simulink model "substation"  (R2018a)
settings: Solver=ode15s  StartTime=0.0  StopTime=0.5  MaxStep=50e-6  RelTol=1e-3  EnableMultiTasking=on
undefined symbols (not defined in the file or in its folder): D1, Delta, Ts
libraries: powerlib x69, powerlib_extras x50
(part 1 of 2)
settings Model: Creator=anton  LastModifiedBy=thain
settings OptimizationCC: LifeSpan=inf
settings DebuggingCC: SFUnexpectedBacktrackingDiag=warning  SFNoUnconditionalDefaultTransitionDiag=warning
settings CodeAppCC: StateflowObjectComments=on
settings GRTTargetCC: TargetLangStandard=C89/C90 (ANSI)
settings ConfigComp: CovMetricSettings=dw  CovSaveCumulativeToWorkspaceVar=on  CovSaveSingleToWorkspaceVar=on  CovExternalEMLEnable=off
settings SimscapeCC: SimscapeNormalizeSystem=off

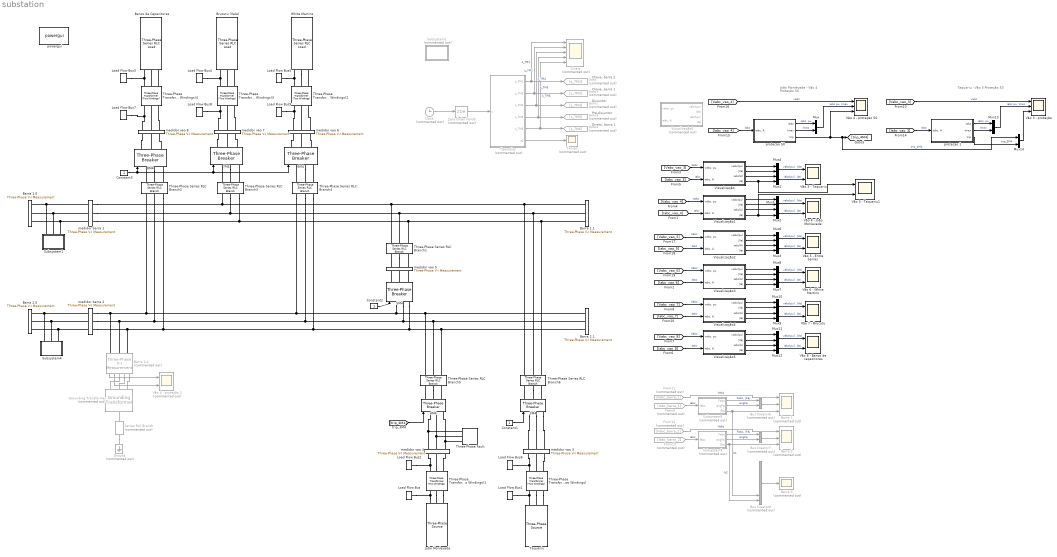
== system substation ==
  note: João Monlevade - Vão 4
      | Proteção 50
  note: Chave, barra 2
  note: Disjuntor
  note: Pré-disjuntor
  note: Chave, barra 1
  note: Direto, barra 1
  note: Taquariu - Vão 3
      | Proteção 50
  3M4 : powerlib/Elements/Three-Phase Breaker  InitialState=closed  SwitchA=on  SwitchB=on  SwitchC=on  SwitchTimes="[1/60  5/60]"  External=on  BreakerResistance=0.01  SnubberResistance=1e6  SnubberCapacitance=inf  Measurements=None
  4M4 : powerlib/Elements/Three-Phase Breaker  InitialState=closed  SwitchA=on  SwitchB=on  SwitchC=on  SwitchTimes="[1/60  5/60]"  External=on  BreakerResistance=0.01  SnubberResistance=1e6  SnubberCapacitance=inf  Measurements=None
  5M4 : powerlib/Elements/Three-Phase Breaker  InitialState=closed  SwitchA=on  SwitchB=on  SwitchC=on  SwitchTimes="[1/60  5/60]"  External=on  BreakerResistance=0.01  SnubberResistance=1e6  SnubberCapacitance=inf  Measurements=None
  6M4 : powerlib/Elements/Three-Phase Breaker  InitialState=closed  SwitchA=on  SwitchB=on  SwitchC=on  SwitchTimes="[1/60  5/60]"  External=on  BreakerResistance=0.01  SnubberResistance=1e6  SnubberCapacitance=inf  Measurements=None
  7M4 : powerlib/Elements/Three-Phase Breaker  InitialState=closed  SwitchA=on  SwitchB=on  SwitchC=on  SwitchTimes="[1/60  5/60]"  External=on  BreakerResistance=0.01  SnubberResistance=1e6  SnubberCapacitance=inf  Measurements=None
  8M4 : powerlib/Elements/Three-Phase Breaker  InitialState=closed  SwitchA=on  SwitchB=on  SwitchC=on  SwitchTimes="[1/60  5/60]"  External=on  BreakerResistance=0.01  SnubberResistance=1e6  SnubberCapacitance=inf  Measurements=None
  Banco de Capacitores : powerlib/Elements/Three-Phase Series RLC Load  LConnTagsString=A|B|C  Configuration=Y (grounded)  NominalVoltage=230e3  Vabc=[1e3 1e3 1e3]  Vabcp=[1e3 1e3 1e3]  NominalFrequency=60  UnbalancedPower=off  ActivePower=capacitor.P  InductivePower=capacitor.QL  CapacitivePower=capacitor.QC  Pabc=[10e3 9e3 11e3]  QLabc=[100 90 110]  QCabc=[100 90 110]  Pabcp=[10e3 9e3 11e3]  QLabcp=[100 90 110]  QCabcp=[100 90 110]  Measurements=None  LoadType=constant Z
  Barra 1 : Scope  Commented=on  NumInputPorts=3
  Barra 1.0 : powerlib/Measurements/Three-Phase V-I Measurement  VoltageMeasurement=no  SetLabelV=off  LabelV=Vabc  Vpu=off  VpuLL=off  CurrentMeasurement=no  SetLabelI=off  LabelI=Iabc  Ipu=off  Pbase=100e6  Vbase=500e3  OutputType=Complex  PhasorSimulation=off  PSBequivalent=0
  Barra 1.1 : powerlib/Measurements/Three-Phase V-I Measurement  VoltageMeasurement=no  SetLabelV=off  LabelV=Vabc  Vpu=off  VpuLL=off  CurrentMeasurement=no  SetLabelI=off  LabelI=Iabc  Ipu=off  Pbase=100e6  Vbase=500e3  OutputType=Complex  PhasorSimulation=off  PSBequivalent=0
  Barra 2 : Scope  Commented=on  NumInputPorts=3
  Barra 2.0 : powerlib/Measurements/Three-Phase V-I Measurement  VoltageMeasurement=no  SetLabelV=off  LabelV=Vabc  Vpu=off  VpuLL=off  CurrentMeasurement=no  SetLabelI=off  LabelI=Iabc  Ipu=off  Pbase=100e6  Vbase=500e3  OutputType=Complex  PhasorSimulation=off  PSBequivalent=0
  Barra 2.1 : powerlib/Measurements/Three-Phase V-I Measurement  VoltageMeasurement=no  SetLabelV=off  LabelV=Vabc  Vpu=off  VpuLL=off  CurrentMeasurement=no  SetLabelI=off  LabelI=Iabc  Ipu=off  Pbase=100e6  Vbase=500e3  OutputType=Complex  PhasorSimulation=off  PSBequivalent=0
  Barra 2.2 : powerlib/Measurements/Three-Phase V-I Measurement  Commented=on  VoltageMeasurement=phase-to-ground  SetLabelV=off  LabelV=Vabc  Vpu=off  VpuLL=off  CurrentMeasurement=yes  SetLabelI=off  LabelI=Iabc  Ipu=off  Pbase=100e6  Vbase=500e3  OutputType=Complex  PhasorSimulation=off  PSBequivalent=0
  Barra 3 : Scope  Commented=on
  Brucutu (Vale) : powerlib/Elements/Three-Phase Series RLC Load  LConnTagsString=A|B|C  Configuration=Y (grounded)  NominalVoltage=230e3  Vabc=[1e3 1e3 1e3]  Vabcp=[1e3 1e3 1e3]  NominalFrequency=60  UnbalancedPower=off  ActivePower=brucutu.P  InductivePower=brucutu.QL  CapacitivePower=brucutu.QC  Pabc=[10e3 9e3 11e3]  QLabc=[100 90 110]  QCabc=[100 90 110]  Pabcp=[10e3 9e3 11e3]  QLabcp=[100 90 110]  QCabcp=[100 90 110]  Measurements=None  LoadType=constant Z
  Bus Creator6 : BusCreator  Commented=on  Inputs=2
  Bus Creator7 : BusCreator  Commented=on  Inputs=2
  Bus Creator8 : BusCreator  Commented=on  Inputs=8
  Clock : Clock  Commented=on
  Constant1 : Constant
  Constant2 : Constant
  Constant3 : Constant
  From11 : From  Commented=on  GotoTag=Vabc_barra_1  TagVisibility=global
  From12 : From  Commented=on  GotoTag=Vabc_barra_2  TagVisibility=global
  From13 : From  Commented=on  GotoTag=Iabc_barra_2  TagVisibility=global
  From9 : From  Commented=on  GotoTag=Iabc_barra_1  TagVisibility=global
  Goto : Goto  Commented=on  GotoTag=s_7M1
  Goto1 : Goto  Commented=on  GotoTag=s_7M2
  Goto2 : Goto  Commented=on  GotoTag=s_7M4
  Goto3 : Goto  Commented=on  GotoTag=s_7M5
  Goto4 : Goto  Commented=on  GotoTag=s_7M6
  Ground : powerlib/Elements/Ground  Commented=on  LConnTagsString=a
  "Grounding Transformer " : powerlib/Elements/Grounding Transformer   Commented=on  UNITS=pu  NominalPower="[1000*100e6   60]"  NominalVoltage=230e3  ZeroSequenceImpedance_pu=[1e-4 1e-4]  MagnetizationBranch_pu=[1e4 1e4]  ZeroSequenceImpedance_SI=[0.052083 589.05]  MagnetizationBranch_SI=[1041.7 3.927e+005]  Measurements=None
      settings: SourceProductName=Simscape Power Systems  SourceProductBaseCode=PS
  João Monlevade : powerlib/Electrical Sources/Three-Phase Source  InternalConnection=Yg  VoltagePhases=off  Voltage=(230000)*1  PhaseAngle=0.0008361  Voltage_phases=[25e3 25e3 25e3]/sqrt(3)  PhaseAngles_phases=[0 -120 +120]  Frequency=60  NonIdealSource=on  SpecifyImpedance=on  Resistance=0  Inductance=0  ShortCircuitLevel=136243*1e6  BaseVoltage=230e3  XRratio=7  BusType=PQ  Pref=monlevade.P  Qref=monlevade.Q  Prefabc=[10e3, 10e3, 10e3]  Qrefabc=[0, 0, 0]  Qmin=-inf  Qmax=inf
  Load Flow Bus : powerlib/Measurements/Load Flow Bus  LConnTagsString=a  Phases=single  Connectors=on one side  ID=BUS_vao4  Vbase=230e3  Vref=1  Vangle=0  VLF=1  VLFb=1  VLFc=1  angleLF=1.025e-06  angleLFb=0  angleLFc=0
      settings: SourceProductName=Simscape Power Systems
  Load Flow Bus1 : powerlib/Measurements/Load Flow Bus  LConnTagsString=a  Phases=single  Connectors=on one side  ID=BUS_vao3  Vbase=230e3  Vref=1  Vangle=0  VLF=1  VLFb=1  VLFc=1  angleLF=0  angleLFb=0  angleLFc=0
      settings: SourceProductName=Simscape Power Systems
  Load Flow Bus2 : powerlib/Measurements/Load Flow Bus  LConnTagsString=a  Phases=single  Connectors=on one side  ID=BUS_vao4_barra  Vbase=230e3  Vref=1  Vangle=0  VLF=1  VLFb=1  VLFc=1  angleLF=-30  angleLFb=0  angleLFc=0
      settings: SourceProductName=Simscape Power Systems
  Load Flow Bus3 : powerlib/Measurements/Load Flow Bus  LConnTagsString=a  Phases=single  Connectors=on one side  ID=BUS_capacitor  Vbase=230e3  Vref=1  Vangle=0  VLF=1  VLFb=1  VLFc=1  angleLF=-7.41e-06  angleLFb=0  angleLFc=0
      settings: SourceProductName=Simscape Power Systems
  Load Flow Bus4 : powerlib/Measurements/Load Flow Bus  LConnTagsString=a  Phases=single  Connectors=on one side  ID=BUS_c2  Vbase=230e3  Vref=1  Vangle=0  VLF=1  VLFb=1  VLFc=1  angleLF=8.861e-06  angleLFb=0  angleLFc=0
      settings: SourceProductName=Simscape Power Systems
  Load Flow Bus5 : powerlib/Measurements/Load Flow Bus  LConnTagsString=a  Phases=single  Connectors=on one side  ID=BUS_c1  Vbase=230e3  Vref=1  Vangle=0  VLF=1  VLFb=1  VLFc=1  angleLF=6.428e-06  angleLFb=0  angleLFc=0
      settings: SourceProductName=Simscape Power Systems
  Load Flow Bus6 : powerlib/Measurements/Load Flow Bus  LConnTagsString=a  Phases=single  Connectors=on one side  ID=BUS_vao3_barra  Vbase=230e3  Vref=1  Vangle=0  VLF=1  VLFb=1  VLFc=1  angleLF=-30  angleLFb=0  angleLFc=0
      settings: SourceProductName=Simscape Power Systems
  Load Flow Bus7 : powerlib/Measurements/Load Flow Bus  LConnTagsString=a  Phases=single  Connectors=on one side  ID=BUS_capacitor_barra  Vbase=230e3  Vref=1  Vangle=0  VLF=1  VLFb=1  VLFc=1  angleLF=-30  angleLFb=0  angleLFc=0
      settings: SourceProductName=Simscape Power Systems
  Load Flow Bus8 : powerlib/Measurements/Load Flow Bus  LConnTagsString=a  Phases=single  Connectors=on one side  ID=BUS_c2_barra  Vbase=230e3  Vref=1  Vangle=0  VLF=1  VLFb=1  VLFc=1  angleLF=-30  angleLFb=0  angleLFc=0
      settings: SourceProductName=Simscape Power Systems
  Load Flow Bus9 : powerlib/Measurements/Load Flow Bus  LConnTagsString=a  Phases=single  Connectors=on one side  ID=BUS_c1_barra  Vbase=230e3  Vref=1  Vangle=0  VLF=1  VLFb=1  VLFc=1  angleLF=-30  angleLFb=0  angleLFc=0
      settings: SourceProductName=Simscape Power Systems
  Mux{,1..14} (15 alike) : Mux  Inputs=2
  Operation : MATLAB Function  Commented=on  TreatAsAtomicUnit=on
  Series RLC Branch : powerlib/Elements/Series RLC Branch  Commented=on  LConnTagsString=__new0  RConnTagsString=__new0  BranchType=R  Resistance=1e12  Inductance=1e-3  SetiL0=off  InitialCurrent=0  Capacitance=1e-6  Setx0=off  InitialVoltage=0  Measurements=None
  Sinais : Scope  Commented=on  NumInputPorts=5
  Subsystem1 : Subsystem
  Subsystem2 : Subsystem  Commented=on
  Subsystem4 : Subsystem
  Subsystem8 : Subsystem  Commented=on
  Subsystem9 : Subsystem  Commented=on
  Taquariu : powerlib/Electrical Sources/Three-Phase Source  InternalConnection=Yg  VoltagePhases=off  Voltage=(230000)*1.00001  PhaseAngle=0.00049007  Voltage_phases=[25e3 25e3 25e3]/sqrt(3)  PhaseAngles_phases=[0 -120 +120]  Frequency=60  NonIdealSource=on  SpecifyImpedance=on  Resistance=0  Inductance=0  ShortCircuitLevel=51788*1e6  BaseVoltage=230e3  XRratio=7  BusType=swing  Pref=11e6  Qref=0  Prefabc=[10e3, 10e3, 10e3]  Qrefabc=[0, 0, 0]  Qmin=-inf  Qmax=inf
  Tempo : Scope  Commented=on
  Three-Phase Series RLC Branch{1..6} (6 alike) : powerlib/Elements/Three-Phase Series RLC Branch  LConnTagsString=A|B|C  RConnTagsString=A|B|C  BranchType=R  Resistance=1e-5  Inductance=1e-3  Capacitance=1e-6  Measurements=None
  Three-Phase Transformer (Two Windings){,1..4} (5 alike) : powerlib/Elements/Three-Phase Transformer (Two Windings)  Winding1Connection=Delta (D1)  Winding2Connection=Yg  CoreType=Three single-phase transformers  SetSaturation=off  Hysteresis=off  DataFile='hysteresis'  SetInitialFlux=off  Measurements=None  UNITS=pu  NominalPower=[ 100e9 , 60 ]  Winding1=[230e3 1e-4 1e-4]  Winding2=[230e3 1e-4 1e-4]  Rm=1e6  Lm=1e6  L0=0.5  Saturation=[0 0;1.8776e-06 3.8348;0.0007823 4.8574]  InitialFluxes=[ 0.8 , -0.8 , 0.7 ]  MoreParameters=off  BreakLoop=off  DataType=off  TransfoNumber=1
  Three-Phase Fault : powerlib/Elements/Three-Phase Fault  InitialStates=0  FaultA=on  FaultB=on  FaultC=on  GroundFault=on  SwitchTimes="[0.1  2+1/60]"  External=off  SwitchStatus=NaN  FaultResistance=0.001  GroundResistance=0.01  SnubberResistance=1e6  SnubberCapacitance=inf  Measurements=None
  Visualização : Subsystem
  Visualização1 : Subsystem
  Visualização2 : Subsystem
  Visualização3 : Subsystem
  Visualização4 : Subsystem
  Visualização5 : Subsystem
  Visualização6 : Subsystem  Commented=on  mask{I_base=2.236}
      mask prompts: I_base "Ibase, A"
  Vão 3 - Taquariu : Scope  NumInputPorts=2
  Vão 3 - Taquariu1 : Scope  NumInputPorts=2
  Vão 3 - proteção : Scope  NumInputPorts=3
  Vão 4 - João Monlevade : Scope  NumInputPorts=2
  Vão 4 - proteção 1 : Scope  Commented=on  NumInputPorts=2
  Vão 4 - proteção 50 : Scope  NumInputPorts=3
  Vão 5 - Entre barras : Scope  NumInputPorts=2
  Vão 6 - White Martins : Scope  NumInputPorts=2
  Vão 7 - Brucutu : Scope  NumInputPorts=2
  Vão 8 - Banco de capacitores : Scope  NumInputPorts=2
  White Martins : powerlib/Elements/Three-Phase Series RLC Load  LConnTagsString=A|B|C  Configuration=Y (grounded)  NominalVoltage=230e3  Vabc=[1e3 1e3 1e3]  Vabcp=[1e3 1e3 1e3]  NominalFrequency=60  UnbalancedPower=off  ActivePower=white.P  InductivePower=white.QL  CapacitivePower=white.QC  Pabc=[10e3 9e3 11e3]  QLabc=[100 90 110]  QCabc=[100 90 110]  Pabcp=[10e3 9e3 11e3]  QLabcp=[100 90 110]  QCabcp=[100 90 110]  Measurements=None  LoadType=constant Z
  Zero-Order Hold3 : ZeroOrderHold  Commented=on  SampleTime=Ts
  medidor barra 1 : powerlib/Measurements/Three-Phase V-I Measurement  VoltageMeasurement=phase-to-ground  SetLabelV=on  LabelV=Vabc_barra_1  Vpu=on  VpuLL=off  CurrentMeasurement=no  SetLabelI=on  LabelI=Iabc_barra_1  Ipu=on  Pbase=16*100e6  Vbase=230e3  OutputType=Complex  PhasorSimulation=off  PSBequivalent=0
  medidor barra 2 : powerlib/Measurements/Three-Phase V-I Measurement  VoltageMeasurement=phase-to-ground  SetLabelV=on  LabelV=Vabc_barra_2  Vpu=on  VpuLL=off  CurrentMeasurement=no  SetLabelI=on  LabelI=Iabc_barra_2  Ipu=off  Pbase=100e6  Vbase=230e3  OutputType=Complex  PhasorSimulation=off  PSBequivalent=0
  medidor vao 3 : powerlib/Measurements/Three-Phase V-I Measurement  VoltageMeasurement=phase-to-ground  SetLabelV=on  LabelV=Vabc_vao_3  Vpu=on  VpuLL=off  CurrentMeasurement=yes  SetLabelI=on  LabelI=Iabc_vao_3  Ipu=off  Pbase=16*100e6  Vbase=230e3  OutputType=Complex  PhasorSimulation=off  PSBequivalent=0
  medidor vao 4 : powerlib/Measurements/Three-Phase V-I Measurement  VoltageMeasurement=phase-to-ground  SetLabelV=on  LabelV=Vabc_vao_4  Vpu=on  VpuLL=off  CurrentMeasurement=yes  SetLabelI=on  LabelI=Iabc_vao_4  Ipu=off  Pbase=16*100e6  Vbase=230e3  OutputType=Complex  PhasorSimulation=off  PSBequivalent=0
  medidor vao 5 : powerlib/Measurements/Three-Phase V-I Measurement  VoltageMeasurement=phase-to-ground  SetLabelV=on  LabelV=Vabc_vao_5  Vpu=on  VpuLL=off  CurrentMeasurement=yes  SetLabelI=on  LabelI=Iabc_vao_5  Ipu=off  Pbase=16*100e6  Vbase=230e3  OutputType=Complex  PhasorSimulation=off  PSBequivalent=0
  medidor vao 6 : powerlib/Measurements/Three-Phase V-I Measurement  VoltageMeasurement=phase-to-ground  SetLabelV=on  LabelV=Vabc_vao_6  Vpu=on  VpuLL=off  CurrentMeasurement=yes  SetLabelI=on  LabelI=Iabc_vao_6  Ipu=off  Pbase=16*100e6  Vbase=230e3  OutputType=Complex  PhasorSimulation=off  PSBequivalent=0
  medidor vao 7 : powerlib/Measurements/Three-Phase V-I Measurement  VoltageMeasurement=phase-to-ground  SetLabelV=on  LabelV=Vabc_vao_7  Vpu=on  VpuLL=off  CurrentMeasurement=yes  SetLabelI=on  LabelI=Iabc_vao_7  Ipu=off  Pbase=16*100e6  Vbase=230e3  OutputType=Complex  PhasorSimulation=off  PSBequivalent=0
  medidor vao 8 : powerlib/Measurements/Three-Phase V-I Measurement  VoltageMeasurement=phase-to-ground  SetLabelV=on  LabelV=Vabc_vao_8  Vpu=on  VpuLL=off  CurrentMeasurement=yes  SetLabelI=on  LabelI=Iabc_vao_8  Ipu=off  Pbase=16*100e6  Vbase=230e3  OutputType=Complex  PhasorSimulation=off  PSBequivalent=0
  powergui : powerlib/powergui  Priority=1  SimulationMode=Discrete  SampleTime=25e-6  frequency=60  Iterations=50  frequencyindice=60  Pbase=100e6  ErrMax=0.0001  UnitsV=kV  UnitsW=MW  buscounter=4  FunctionMessages=off  echomessages=off  EnableUseOfTLC=off  CurrentSourceSwitches=off  DisableSnubberDevices=off  DisableRonSwitches=off  DisableVfSwitches=off  DisplayEquations=off  SolverType=Tustin/Backward Euler (TBE)  Interpol=off  ExternalGateDelay=off  methode=off  Ts=100  x0status=blocks  SPID=off  SwTol=0  HookPort=off  RestoreLinks=warning  ResistiveCurrentMeasurement=off  Frange=[0:2:500]  Ylog=off  Xlog=on  ShowGrid=off  save=off  variable=ZData  structure=0  ZoomFFT=off  StartTime=0.0  cycles=1  DisplayStyle=1  fundamental=60  FreqAxis=off  MaxFrequency=1000  frequencyindicesteady=1  RmsSteady=1  display=off
  protecao 1 : Subsystem  mask{Ipick_up=0*6.8 + 4.8e5/2, td_op=1.0*(1/60)}
      mask prompts: Ipick_up "Ipick-up, A"; td_op "delay de operação, s"
  protecao 50 : Subsystem  mask{Ipick_up=0*6.8 + 4.8e5/2, td_op=1.0*(1/60)}
      mask prompts: Ipick_up "Ipick-up, A"; td_op "delay de operação, s"
  wires:
  Operation/5(s_7M6) -> Sinais/5, Goto4/1  "s_7M6"
  Operation/6(t0) -> Tempo/1
  Operation/4(s_7M5) -> Sinais/4, Goto3/1  "s_7M5"
  Operation/2(s_7M2) -> Sinais/2, Goto1/1  "s_7M2"
  Zero-Order Hold3/1 -> Operation/1(t)
  Operation/3(s_7M4) -> Sinais/3, Goto2/1  "s_7M4"
  Clock/1 -> Zero-Order Hold3/1
  Operation/1(s_7M1) -> Sinais/1, Goto/1  "s_7M1"
  Constant2/1 -> 5M4/1
  Constant3/1 -> 6M4/1, 7M4/1, 8M4/1
  Bus Creator6/1 -> Barra 1/2
  Subsystem8/3(|Fa|) -> Bus Creator8/7, Barra 1/3  "b1"
  Subsystem8/2(angFa) -> Bus Creator6/2  "angFa"
  Subsystem8/1(Fabc) -> Bus Creator6/1  "Fabc, |Fa|"
  From9/1 -> Subsystem8/1(fabc)  "Iabc"
  From11/1 -> Barra 1/1  "Vabc"
  From12/1 -> Barra 2/1  "Vabc"
  From13/1 -> Subsystem9/1(fabc)  "Iabc"
  Subsystem9/1(Fabc) -> Bus Creator7/1  "Fabc, |Fa|"
  Subsystem9/2(angFa) -> Bus Creator7/2  "angFa"
  Subsystem9/3(|Fa|) -> Bus Creator8/8, Barra 2/3  "b2"
  Bus Creator7/1 -> Barra 2/2
  Bus Creator8/1 -> Barra 3/1
  protecao 50/3(trip) -> Mux14/1, [trip_4M4], Vão 4 - proteção 50/3  "trip_4M4"
  protecao 50/1(iabc) -> Mux/1  "iabc, pu"
  Mux/1 -> Vão 4 - proteção 50/2  "iabc pu, Imax"
  [Iabc_vao_4] -> protecao 50/1("iabc, A")  "Iabc"
  protecao 50/2(Imax) -> Mux/2  "Imax"
  [Vabc_vao_4] -> Vão 4 - proteção 50/1  "vabc"
  [Vabc_vao_3] -> Visualização/1("vabc, pu")  "Vabc"
  [Iabc_vao_3] -> Visualização/2("iabc, A")  "Iabc"
  Mux4/1 -> Vão 3 - Taquariu/1  "vabc(pu), |Va|"
  Mux1/1 -> Vão 3 - Taquariu/2  "iabc(pu), |Ia|"
  Visualização/4(|Ia|) -> Vão 3 - Taquariu1/1, Mux1/2
  Visualização/3(iabc(A)) -> Mux1/1
  [Iabc_vao_4] -> Visualização1/2("iabc, A")  "Iabc"
  [Vabc_vao_4] -> Visualização1/1("vabc, pu")  "Vabc"
  [Vabc_vao_5] -> Visualização2/1("vabc, pu")  "Vabc"
  [Iabc_vao_5] -> Visualização2/2("iabc, A")  "Iabc"
  Visualização/1(vabc(pu)) -> Mux4/1
  Visualização/2(|Va|) -> Mux4/2
  Visualização1/2(|Va|) -> Mux5/2
  Visualização1/1(vabc(pu)) -> Mux5/1
  Visualização1/3(iabc(A)) -> Mux2/1
  Visualização1/4(|Ia|) -> Vão 3 - Taquariu1/2, Mux2/2
  Mux2/1 -> Vão 4 - João Monlevade/2  "iabc(pu), |Ia|"
  Mux5/1 -> Vão 4 - João Monlevade/1  "vabc(pu), |Va|"
  Mux6/1 -> Vão 5 - Entre barras/1  "vabc(pu), |Va|"
  Mux3/1 -> Vão 5 - Entre barras/2  "iabc(pu), |Ia|"
  Visualização2/4(|Ia|) -> Mux3/2
  Visualização2/3(iabc(A)) -> Mux3/1
  Visualização2/1(vabc(pu)) -> Mux6/1
  Visualização2/2(|Va|) -> Mux6/2
  Visualização3/2(|Va|) -> Mux8/2
  Visualização3/1(vabc(pu)) -> Mux8/1
  Visualização3/3(iabc(A)) -> Mux7/1
  Visualização3/4(|Ia|) -> Mux7/2
  Mux7/1 -> Vão 6 - White Martins/2  "iabc(pu), |Ia|"
  Mux8/1 -> Vão 6 - White Martins/1  "vabc(pu), |Va|"
  [Iabc_vao_6] -> Visualização3/2("iabc, A")  "Iabc"
  [Vabc_vao_6] -> Visualização3/1("vabc, pu")  "Vabc"
  [Vabc_vao_7] -> Visualização4/1("vabc, pu")  "Vabc"
  [Iabc_vao_7] -> Visualização4/2("iabc, A")  "Iabc"
  Mux10/1 -> Vão 7 - Brucutu/1  "vabc(pu), |Va|"
  Mux9/1 -> Vão 7 - Brucutu/2  "iabc(pu), |Ia|"
  Visualização4/4(|Ia|) -> Mux9/2
  Visualização4/3(iabc(A)) -> Mux9/1
  Visualização4/1(vabc(pu)) -> Mux10/1
  Visualização4/2(|Va|) -> Mux10/2
  Visualização5/2(|Va|) -> Mux11/2
  Visualização5/1(vabc(pu)) -> Mux11/1
  Visualização5/3(iabc(A)) -> Mux12/1
  Visualização5/4(|Ia|) -> Mux12/2
  Mux12/1 -> Vão 8 - Banco de capacitores/2  "iabc(pu), |Ia|"
  Mux11/1 -> Vão 8 - Banco de capacitores/1  "vabc(pu), |Va|"
  [Iabc_vao_8] -> Visualização5/2("iabc, A")  "Iabc"
  [Vabc_vao_8] -> Visualização5/1("vabc, pu")  "Vabc"
  Barra 2.2/1 -> Vão 4 - proteção 1/1
  Barra 2.2/2 -> Vão 4 - proteção 1/2
  Constant1/1 -> 3M4/1
  [trip_4M4] -> 4M4/1
  [Vabc_vao_3] -> Vão 3 - proteção/1  "vabc"
  protecao 1/2(Imax) -> Mux13/2  "Imax"
  [Iabc_vao_3] -> protecao 1/1("iabc, A")  "Iabc"
  Mux13/1 -> Vão 3 - proteção/2  "iabc pu, Imax"
  protecao 1/1(iabc) -> Mux13/1  "iabc, pu"
  protecao 1/3(trip) -> Mux14/2  "trip_3M4"
  Mux14/1 -> Vão 3 - proteção/3
  connections:
  medidor barra 2/RConn3 -- Barra 2.2/LConn3 -- Three-Phase Series RLC Branch2/LConn3 -- Three-Phase Series RLC Branch4/LConn3 -- 5M4/LConn3 -- Barra 2.1/LConn3 -- Three-Phase Series RLC Branch5/RConn3
  5M4/RConn1 -- medidor vao 5/RConn1
  5M4/RConn2 -- medidor vao 5/RConn2
  5M4/RConn3 -- medidor vao 5/RConn3
  medidor barra 1/LConn3 -- Subsystem1/LConn3 -- Barra 1.0/RConn3
  medidor barra 1/LConn2 -- Subsystem1/LConn2 -- Barra 1.0/RConn2
  medidor barra 1/LConn1 -- Subsystem1/LConn1 -- Barra 1.0/RConn1
  medidor barra 2/LConn3 -- Subsystem4/LConn3 -- Barra 2.0/RConn3
  medidor barra 2/LConn2 -- Subsystem4/LConn2 -- Barra 2.0/RConn2
  Load Flow Bus2/LConn1 -- medidor vao 4/RConn1 -- Three-Phase Transformer (Two Windings)1/LConn1
  Load Flow Bus6/LConn1 -- medidor vao 3/RConn1 -- Three-Phase Transformer (Two Windings)/LConn1
  Three-Phase Transformer (Two Windings)/RConn2 -- Taquariu/RConn2
  Taquariu/RConn1 -- Three-Phase Transformer (Two Windings)/RConn1 -- Load Flow Bus1/LConn1
  Three-Phase Transformer (Two Windings)/RConn3 -- Taquariu/RConn3
  João Monlevade/RConn1 -- Three-Phase Transformer (Two Windings)1/RConn1 -- Load Flow Bus/LConn1
  Three-Phase Transformer (Two Windings)1/RConn2 -- João Monlevade/RConn2
  Three-Phase Transformer (Two Windings)1/RConn3 -- João Monlevade/RConn3
  Three-Phase Transformer (Two Windings)2/RConn1 -- Load Flow Bus5/LConn1 -- White Martins/LConn1
  White Martins/LConn2 -- Three-Phase Transformer (Two Windings)2/RConn2
  Three-Phase Transformer (Two Windings)2/RConn3 -- White Martins/LConn3
  Load Flow Bus9/LConn1 -- medidor vao 6/LConn1 -- Three-Phase Transformer (Two Windings)2/LConn1
  Three-Phase Transformer (Two Windings)3/RConn2 -- Brucutu (Vale)/LConn2
  Three-Phase Transformer (Two Windings)3/RConn1 -- Load Flow Bus4/LConn1 -- Brucutu (Vale)/LConn1
  Three-Phase Transformer (Two Windings)3/RConn3 -- Brucutu (Vale)/LConn3
  Load Flow Bus8/LConn1 -- medidor vao 7/LConn1 -- Three-Phase Transformer (Two Windings)3/LConn1
  Three-Phase Transformer (Two Windings)4/RConn2 -- Banco de Capacitores/LConn2
  Three-Phase Transformer (Two Windings)4/RConn1 -- Load Flow Bus3/LConn1 -- Banco de Capacitores/LConn1
  Three-Phase Transformer (Two Windings)4/RConn3 -- Banco de Capacitores/LConn3
  Load Flow Bus7/LConn1 -- medidor vao 8/LConn1 -- Three-Phase Transformer (Two Windings)4/LConn1
  medidor barra 2/RConn1 -- Barra 2.2/LConn1 -- Three-Phase Series RLC Branch2/LConn1 -- Three-Phase Series RLC Branch4/LConn1 -- 5M4/LConn1 -- Barra 2.1/LConn1 -- Three-Phase Series RLC Branch5/RConn1
  medidor barra 2/RConn2 -- Barra 2.2/LConn2 -- Three-Phase Series RLC Branch2/LConn2 -- Three-Phase Series RLC Branch4/LConn2 -- 5M4/LConn2 -- Barra 2.1/LConn2 -- Three-Phase Series RLC Branch5/RConn2
  medidor barra 1/RConn1 -- Three-Phase Series RLC Branch3/LConn1 -- Three-Phase Series RLC Branch1/RConn1 -- Three-Phase Series RLC Branch6/RConn1 -- Barra 1.1/LConn1
  medidor barra 1/RConn2 -- Three-Phase Series RLC Branch3/LConn2 -- Three-Phase Series RLC Branch1/RConn2 -- Three-Phase Series RLC Branch6/RConn2 -- Barra 1.1/LConn2
  medidor barra 1/RConn3 -- Three-Phase Series RLC Branch1/RConn3 -- Three-Phase Series RLC Branch6/RConn3 -- Barra 1.1/LConn3 -- Three-Phase Series RLC Branch3/LConn3
  medidor vao 5/LConn1 -- Three-Phase Series RLC Branch1/LConn1
  Three-Phase Series RLC Branch1/LConn2 -- medidor vao 5/LConn2
  medidor vao 5/LConn3 -- Three-Phase Series RLC Branch1/LConn3
  3M4/RConn1 -- Three-Phase Series RLC Branch6/LConn1
  Three-Phase Series RLC Branch6/LConn2 -- 3M4/RConn2
  3M4/RConn3 -- Three-Phase Series RLC Branch6/LConn3
  3M4/LConn2 -- medidor vao 3/LConn2
  3M4/LConn1 -- medidor vao 3/LConn1
  3M4/LConn3 -- medidor vao 3/LConn3
  medidor vao 3/RConn3 -- Three-Phase Transformer (Two Windings)/LConn3
  Three-Phase Transformer (Two Windings)/LConn2 -- medidor vao 3/RConn2
  4M4/RConn1 -- Three-Phase Series RLC Branch5/LConn1
  Three-Phase Series RLC Branch5/LConn2 -- 4M4/RConn2
  4M4/RConn3 -- Three-Phase Series RLC Branch5/LConn3
  medidor vao 4/RConn3 -- Three-Phase Transformer (Two Windings)1/LConn3
  Three-Phase Transformer (Two Windings)1/LConn2 -- medidor vao 4/RConn2
  medidor vao 4/LConn2 -- Three-Phase Fault/LConn2 -- 4M4/LConn2
  medidor vao 4/LConn3 -- Three-Phase Fault/LConn3 -- 4M4/LConn3
  medidor vao 4/LConn1 -- Three-Phase Fault/LConn1 -- 4M4/LConn1
  Three-Phase Series RLC Branch4/RConn1 -- 6M4/LConn1
  6M4/LConn2 -- Three-Phase Series RLC Branch4/RConn2
  Three-Phase Series RLC Branch4/RConn3 -- 6M4/LConn3
  Three-Phase Series RLC Branch3/RConn1 -- 7M4/LConn1
  7M4/LConn2 -- Three-Phase Series RLC Branch3/RConn2
  Three-Phase Series RLC Branch3/RConn3 -- 7M4/LConn3
  Three-Phase Series RLC Branch2/RConn1 -- 8M4/LConn1
  8M4/LConn2 -- Three-Phase Series RLC Branch2/RConn2
  Three-Phase Series RLC Branch2/RConn3 -- 8M4/LConn3
  8M4/RConn2 -- medidor vao 8/RConn2
  8M4/RConn1 -- medidor vao 8/RConn1
  8M4/RConn3 -- medidor vao 8/RConn3
  7M4/RConn2 -- medidor vao 7/RConn2
  7M4/RConn1 -- medidor vao 7/RConn1
  7M4/RConn3 -- medidor vao 7/RConn3
  6M4/RConn2 -- medidor vao 6/RConn2
  6M4/RConn1 -- medidor vao 6/RConn1
  6M4/RConn3 -- medidor vao 6/RConn3
  medidor vao 8/LConn3 -- Three-Phase Transformer (Two Windings)4/LConn3
  medidor vao 8/LConn2 -- Three-Phase Transformer (Two Windings)4/LConn2
  medidor vao 7/LConn3 -- Three-Phase Transformer (Two Windings)3/LConn3
  medidor vao 7/LConn2 -- Three-Phase Transformer (Two Windings)3/LConn2
  medidor vao 6/LConn3 -- Three-Phase Transformer (Two Windings)2/LConn3
  medidor vao 6/LConn2 -- Three-Phase Transformer (Two Windings)2/LConn2
  Barra 2.2/RConn1 -- "Grounding Transformer "/LConn1
  Barra 2.2/RConn2 -- "Grounding Transformer "/LConn2
  Barra 2.2/RConn3 -- "Grounding Transformer "/LConn3
  Series RLC Branch/RConn1 -- Ground/LConn1
  Series RLC Branch/LConn1 -- "Grounding Transformer "/RConn1
  medidor barra 2/LConn1 -- Subsystem4/LConn1 -- Barra 2.0/RConn1

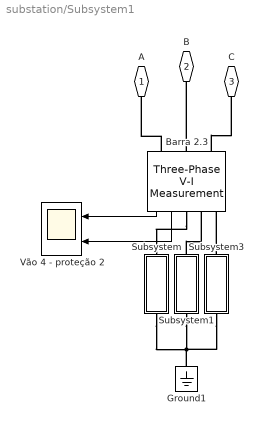
== system substation/Subsystem1 ==
  Barra 2.3 : powerlib/Measurements/Three-Phase V-I Measurement  VoltageMeasurement=phase-to-ground  SetLabelV=off  LabelV=Vabc  Vpu=off  VpuLL=off  CurrentMeasurement=yes  SetLabelI=off  LabelI=Iabc  Ipu=off  Pbase=100e6  Vbase=500e3  OutputType=Complex  PhasorSimulation=off  PSBequivalent=0
  Ground1 : powerlib/Elements/Ground  LConnTagsString=a
  Subsystem : Subsystem
  Subsystem1 : Subsystem
  Subsystem3 : Subsystem
  Vão 4 - proteção 2 : Scope  NumInputPorts=2
  A : PMIOPort  Side=Left
  B : PMIOPort  Port=2  Side=Left
  C : PMIOPort  Port=3  Side=Left
  wires:
  Barra 2.3/1 -> Vão 4 - proteção 2/1
  Barra 2.3/2 -> Vão 4 - proteção 2/2
  connections:
  Barra 2.3/LConn2 -- B/RConn1
  Barra 2.3/LConn3 -- C/RConn1
  Barra 2.3/RConn1 -- Subsystem/LConn1
  Subsystem3/RConn1 -- Ground1/LConn1 -- Subsystem/RConn1 -- Subsystem1/RConn1
  Subsystem1/LConn1 -- Barra 2.3/RConn2
  Subsystem3/LConn1 -- Barra 2.3/RConn3
  Barra 2.3/LConn1 -- A/RConn1

== system substation/Subsystem2 ==
  AC Voltage Source : powerlib/Electrical Sources/AC Voltage Source  Amplitude=sqrt(2)*230e3  Phase=-120  Frequency=60  SampleTime=0  Measurements=None  BusType=swing  Pref=10e3  Qref=0  Qmin=-inf  Qmax=+inf
  AC Voltage Source1 : powerlib/Electrical Sources/AC Voltage Source  Amplitude=sqrt(2)*230e3  Phase=0  Frequency=60  SampleTime=0  Measurements=None  BusType=swing  Pref=10e3  Qref=0  Qmin=-inf  Qmax=+inf
  AC Voltage Source2 : powerlib/Electrical Sources/AC Voltage Source  Amplitude=sqrt(2)*230e3  Phase=120  Frequency=60  SampleTime=0  Measurements=None  BusType=swing  Pref=10e3  Qref=0  Qmin=-inf  Qmax=+inf
  A : PMIOPort  Side=Left
  B : PMIOPort  Port=2  Side=Left
  C : PMIOPort  Port=3  Side=Left
  connections:
  AC Voltage Source1/RConn1 -- A/RConn1 -- AC Voltage Source2/LConn1
  AC Voltage Source/LConn1 -- C/RConn1 -- AC Voltage Source2/RConn1
  AC Voltage Source1/LConn1 -- B/RConn1 -- AC Voltage Source/RConn1

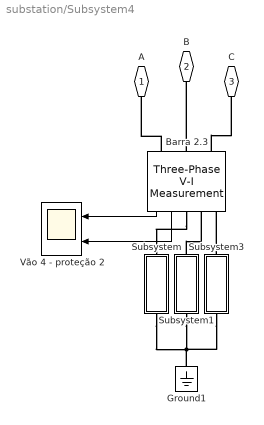
== system substation/Subsystem4 ==
  Barra 2.3 : powerlib/Measurements/Three-Phase V-I Measurement  VoltageMeasurement=phase-to-ground  SetLabelV=off  LabelV=Vabc  Vpu=off  VpuLL=off  CurrentMeasurement=yes  SetLabelI=off  LabelI=Iabc  Ipu=off  Pbase=100e6  Vbase=500e3  OutputType=Complex  PhasorSimulation=off  PSBequivalent=0
  Ground1 : powerlib/Elements/Ground  LConnTagsString=a
  Subsystem : Subsystem
  Subsystem1 : Subsystem
  Subsystem3 : Subsystem
  Vão 4 - proteção 2 : Scope  NumInputPorts=2
  A : PMIOPort  Side=Left
  B : PMIOPort  Port=2  Side=Left
  C : PMIOPort  Port=3  Side=Left
  wires:
  Barra 2.3/2 -> Vão 4 - proteção 2/2
  Barra 2.3/1 -> Vão 4 - proteção 2/1
  connections:
  Barra 2.3/LConn1 -- A/RConn1
  Subsystem3/LConn1 -- Barra 2.3/RConn3
  Subsystem1/LConn1 -- Barra 2.3/RConn2
  Ground1/LConn1 -- Subsystem3/RConn1 -- Subsystem1/RConn1 -- Subsystem/RConn1
  Barra 2.3/RConn1 -- Subsystem/LConn1
  Barra 2.3/LConn3 -- C/RConn1
  Barra 2.3/LConn2 -- B/RConn1

== system substation/Subsystem8 ==
  fabc : Inport
  Demux1 : Demux  Outputs=3
  RMS : powerlib_extras/Measurements/Fourier  f1=60  n=1
  Terminator : Terminator
  Terminator1 : Terminator
  Fabc : Outport
  angFa : Outport  Port=2
  |Fa| : Outport  Port=3
  wires:
  Demux1/2 -> Terminator/1
  Demux1/1 -> RMS/1
  fabc/1 -> Demux1/1, Fabc/1
  RMS/1 -> |Fa|/1  "|fa|"
  RMS/2 -> angFa/1  "angIa"
  Demux1/3 -> Terminator1/1

== system substation/Subsystem9 ==
  fabc : Inport
  Demux1 : Demux  Outputs=3
  RMS : powerlib_extras/Measurements/Fourier  f1=60  n=1
  Terminator : Terminator
  Terminator1 : Terminator
  Fabc : Outport
  angFa : Outport  Port=2
  |Fa| : Outport  Port=3
  wires:
  Demux1/3 -> Terminator1/1
  RMS/2 -> angFa/1  "angIa"
  RMS/1 -> |Fa|/1  "|fa|"
  fabc/1 -> Fabc/1, Demux1/1
  Demux1/1 -> RMS/1
  Demux1/2 -> Terminator/1

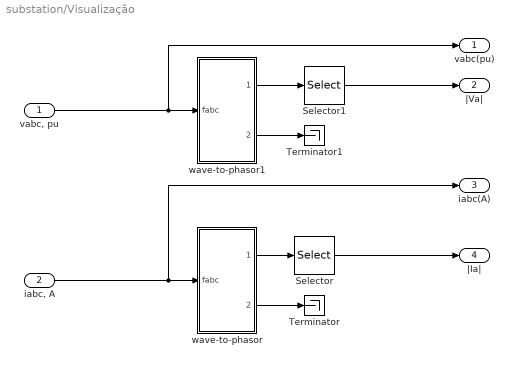
== system substation/Visualização ==
  "vabc, pu" : Inport
  "iabc, A" : Inport  Port=2
  Selector : Selector  InputPortWidth=3  IndexOptions=Index vector (dialog)  Indices=[1]  OutputSizes=1
  Selector1 : Selector  InputPortWidth=3  IndexOptions=Index vector (dialog)  Indices=[1]  OutputSizes=1
  Terminator : Terminator
  Terminator1 : Terminator
  wave-to-phasor : Subsystem
  wave-to-phasor1 : Subsystem
  vabc(pu) : Outport
  |Va| : Outport  Port=2
  iabc(A) : Outport  Port=3
  |Ia| : Outport  Port=4
  wires:
  wave-to-phasor/2(ang(Fabc)) -> Terminator/1
  wave-to-phasor/1(|Fabc|) -> Selector/1
  Selector/1 -> |Ia|/1
  "iabc, A"/1 -> iabc(A)/1, wave-to-phasor/1(fabc)
  "vabc, pu"/1 -> vabc(pu)/1, wave-to-phasor1/1(fabc)
  Selector1/1 -> |Va|/1
  wave-to-phasor1/1(|Fabc|) -> Selector1/1
  wave-to-phasor1/2(ang(Fabc)) -> Terminator1/1

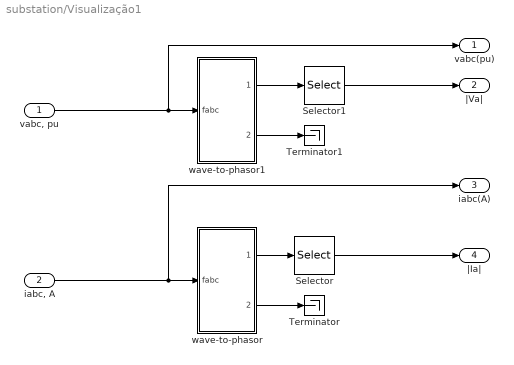
== system substation/Visualização1 ==
  "vabc, pu" : Inport
  "iabc, A" : Inport  Port=2
  Selector : Selector  InputPortWidth=3  IndexOptions=Index vector (dialog)  Indices=[1]  OutputSizes=1
  Selector1 : Selector  InputPortWidth=3  IndexOptions=Index vector (dialog)  Indices=[1]  OutputSizes=1
  Terminator : Terminator
  Terminator1 : Terminator
  wave-to-phasor : Subsystem
  wave-to-phasor1 : Subsystem
  vabc(pu) : Outport
  |Va| : Outport  Port=2
  iabc(A) : Outport  Port=3
  |Ia| : Outport  Port=4
  wires:
  wave-to-phasor1/2(ang(Fabc)) -> Terminator1/1
  wave-to-phasor1/1(|Fabc|) -> Selector1/1
  Selector1/1 -> |Va|/1
  "vabc, pu"/1 -> wave-to-phasor1/1(fabc), vabc(pu)/1
  "iabc, A"/1 -> wave-to-phasor/1(fabc), iabc(A)/1
  Selector/1 -> |Ia|/1
  wave-to-phasor/1(|Fabc|) -> Selector/1
  wave-to-phasor/2(ang(Fabc)) -> Terminator/1

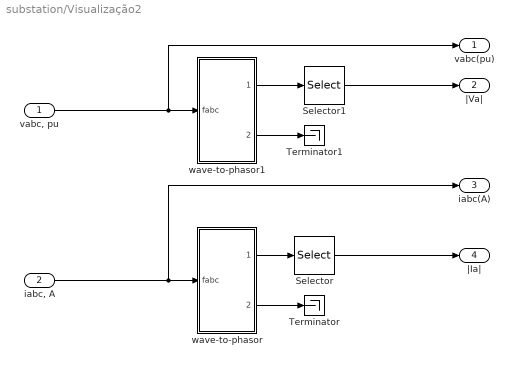
== system substation/Visualização2 ==
  "vabc, pu" : Inport
  "iabc, A" : Inport  Port=2
  Selector : Selector  InputPortWidth=3  IndexOptions=Index vector (dialog)  Indices=[1]  OutputSizes=1
  Selector1 : Selector  InputPortWidth=3  IndexOptions=Index vector (dialog)  Indices=[1]  OutputSizes=1
  Terminator : Terminator
  Terminator1 : Terminator
  wave-to-phasor : Subsystem
  wave-to-phasor1 : Subsystem
  vabc(pu) : Outport
  |Va| : Outport  Port=2
  iabc(A) : Outport  Port=3
  |Ia| : Outport  Port=4
  wires:
  wave-to-phasor/2(ang(Fabc)) -> Terminator/1
  wave-to-phasor/1(|Fabc|) -> Selector/1
  Selector/1 -> |Ia|/1
  "iabc, A"/1 -> iabc(A)/1, wave-to-phasor/1(fabc)
  "vabc, pu"/1 -> vabc(pu)/1, wave-to-phasor1/1(fabc)
  Selector1/1 -> |Va|/1
  wave-to-phasor1/1(|Fabc|) -> Selector1/1
  wave-to-phasor1/2(ang(Fabc)) -> Terminator1/1

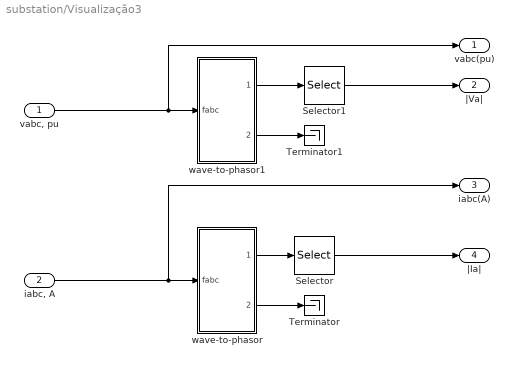
== system substation/Visualização3 ==
  "vabc, pu" : Inport
  "iabc, A" : Inport  Port=2
  Selector : Selector  InputPortWidth=3  IndexOptions=Index vector (dialog)  Indices=[1]  OutputSizes=1
  Selector1 : Selector  InputPortWidth=3  IndexOptions=Index vector (dialog)  Indices=[1]  OutputSizes=1
  Terminator : Terminator
  Terminator1 : Terminator
  wave-to-phasor : Subsystem
  wave-to-phasor1 : Subsystem
  vabc(pu) : Outport
  |Va| : Outport  Port=2
  iabc(A) : Outport  Port=3
  |Ia| : Outport  Port=4
  wires:
  wave-to-phasor1/2(ang(Fabc)) -> Terminator1/1
  wave-to-phasor1/1(|Fabc|) -> Selector1/1
  Selector1/1 -> |Va|/1
  "vabc, pu"/1 -> wave-to-phasor1/1(fabc), vabc(pu)/1
  "iabc, A"/1 -> wave-to-phasor/1(fabc), iabc(A)/1
  Selector/1 -> |Ia|/1
  wave-to-phasor/1(|Fabc|) -> Selector/1
  wave-to-phasor/2(ang(Fabc)) -> Terminator/1

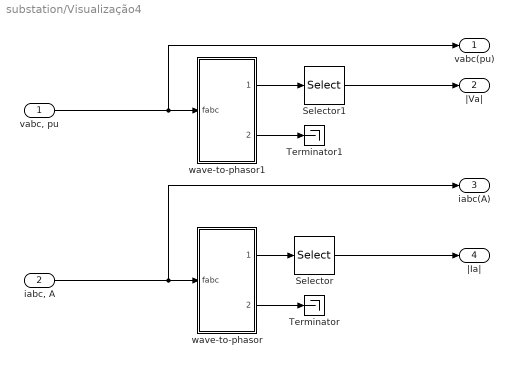
== system substation/Visualização4 ==
  "vabc, pu" : Inport
  "iabc, A" : Inport  Port=2
  Selector : Selector  InputPortWidth=3  IndexOptions=Index vector (dialog)  Indices=[1]  OutputSizes=1
  Selector1 : Selector  InputPortWidth=3  IndexOptions=Index vector (dialog)  Indices=[1]  OutputSizes=1
  Terminator : Terminator
  Terminator1 : Terminator
  wave-to-phasor : Subsystem
  wave-to-phasor1 : Subsystem
  vabc(pu) : Outport
  |Va| : Outport  Port=2
  iabc(A) : Outport  Port=3
  |Ia| : Outport  Port=4
  wires:
  wave-to-phasor/2(ang(Fabc)) -> Terminator/1
  wave-to-phasor/1(|Fabc|) -> Selector/1
  Selector/1 -> |Ia|/1
  "iabc, A"/1 -> iabc(A)/1, wave-to-phasor/1(fabc)
  "vabc, pu"/1 -> vabc(pu)/1, wave-to-phasor1/1(fabc)
  Selector1/1 -> |Va|/1
  wave-to-phasor1/1(|Fabc|) -> Selector1/1
  wave-to-phasor1/2(ang(Fabc)) -> Terminator1/1

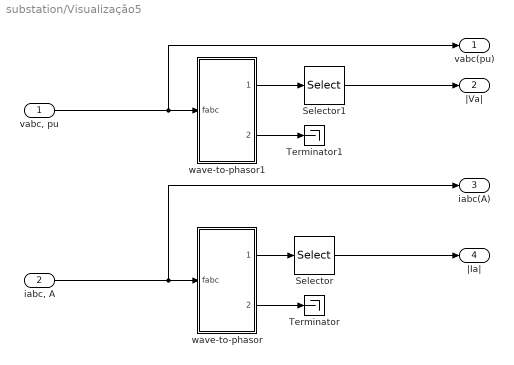
== system substation/Visualização5 ==
  "vabc, pu" : Inport
  "iabc, A" : Inport  Port=2
  Selector : Selector  InputPortWidth=3  IndexOptions=Index vector (dialog)  Indices=[1]  OutputSizes=1
  Selector1 : Selector  InputPortWidth=3  IndexOptions=Index vector (dialog)  Indices=[1]  OutputSizes=1
  Terminator : Terminator
  Terminator1 : Terminator
  wave-to-phasor : Subsystem
  wave-to-phasor1 : Subsystem
  vabc(pu) : Outport
  |Va| : Outport  Port=2
  iabc(A) : Outport  Port=3
  |Ia| : Outport  Port=4
  wires:
  wave-to-phasor1/2(ang(Fabc)) -> Terminator1/1
  wave-to-phasor1/1(|Fabc|) -> Selector1/1
  Selector1/1 -> |Va|/1
  "vabc, pu"/1 -> wave-to-phasor1/1(fabc), vabc(pu)/1
  "iabc, A"/1 -> wave-to-phasor/1(fabc), iabc(A)/1
  Selector/1 -> |Ia|/1
  wave-to-phasor/1(|Fabc|) -> Selector/1
  wave-to-phasor/2(ang(Fabc)) -> Terminator/1

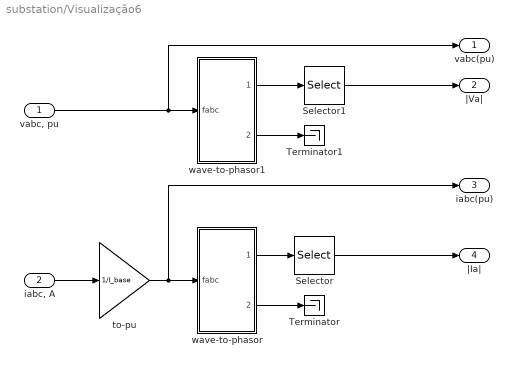
== system substation/Visualização6 ==
  "vabc, pu" : Inport
  "iabc, A" : Inport  Port=2
  Selector : Selector  InputPortWidth=3  IndexOptions=Index vector (dialog)  Indices=[1]  OutputSizes=1
  Selector1 : Selector  InputPortWidth=3  IndexOptions=Index vector (dialog)  Indices=[1]  OutputSizes=1
  Terminator : Terminator
  Terminator1 : Terminator
  to-pu : Gain  Gain=1/I_base
  wave-to-phasor : Subsystem
  wave-to-phasor1 : Subsystem
  vabc(pu) : Outport
  |Va| : Outport  Port=2
  iabc(pu) : Outport  Port=3
  |Ia| : Outport  Port=4
  wires:
  wave-to-phasor1/2(ang(Fabc)) -> Terminator1/1
  wave-to-phasor1/1(|Fabc|) -> Selector1/1
  Selector1/1 -> |Va|/1
  "vabc, pu"/1 -> wave-to-phasor1/1(fabc), vabc(pu)/1
  to-pu/1 -> wave-to-phasor/1(fabc), iabc(pu)/1
  Selector/1 -> |Ia|/1
  "iabc, A"/1 -> to-pu/1
  wave-to-phasor/1(|Fabc|) -> Selector/1
  wave-to-phasor/2(ang(Fabc)) -> Terminator/1

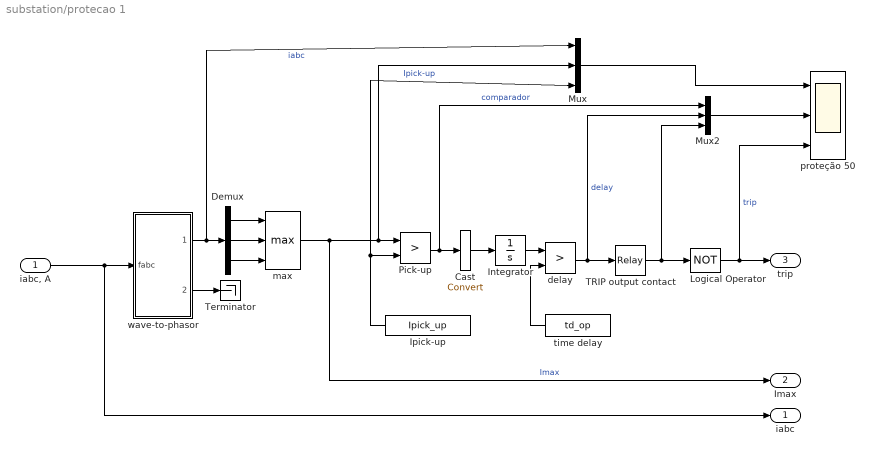
== system substation/protecao 1 ==
  "iabc, A" : Inport
  Cast : DataTypeConversion
  Demux : Demux  Outputs=3
  Integrator : Integrator
  Ipick-up : Constant  Value=Ipick_up
  Logical Operator : Logic  Operator=NOT  Inputs=1
  Mux : Mux  Inputs=3
  Mux2 : Mux  Inputs=3
  Pick-up : RelationalOperator  Operator=>  RndMeth=Nearest  InputSameDT=on
  TRIP output contact : Relay  OnSwitchValue=0.9999  OffSwitchValue=-1
  Terminator : Terminator
  delay : RelationalOperator  Operator=>  RndMeth=Nearest  InputSameDT=on
  max : MinMax  Function=max  Inputs=3
  proteção 50 : Scope  NumInputPorts=3
  time delay : Constant  Value=td_op
  wave-to-phasor : Subsystem
  iabc : Outport
  Imax : Outport  Port=2
  trip : Outport  Port=3
  wires:
  wave-to-phasor/2(ang(Fabc)) -> Terminator/1
  "iabc, A"/1 -> iabc/1, wave-to-phasor/1(fabc)
  wave-to-phasor/1(|Fabc|) -> Demux/1, Mux/1  "iabc"
  Demux/3 -> max/3
  Demux/2 -> max/2
  Demux/1 -> max/1
  Integrator/1 -> delay/1
  Ipick-up/1 -> Pick-up/2, Mux/3  "Ipick-up"
  Pick-up/1 -> Mux2/1, Cast/1  "comparador"
  Mux/1 -> proteção 50/1
  Logical Operator/1 -> proteção 50/3, trip/1  "trip"
  delay/1 -> Mux2/2, TRIP output contact/1  "delay"
  time delay/1 -> delay/2
  Cast/1 -> Integrator/1
  Mux2/1 -> proteção 50/2
  TRIP output contact/1 -> Mux2/3, Logical Operator/1
  max/1 -> Pick-up/1, Mux/2, Imax/1  "Imax"

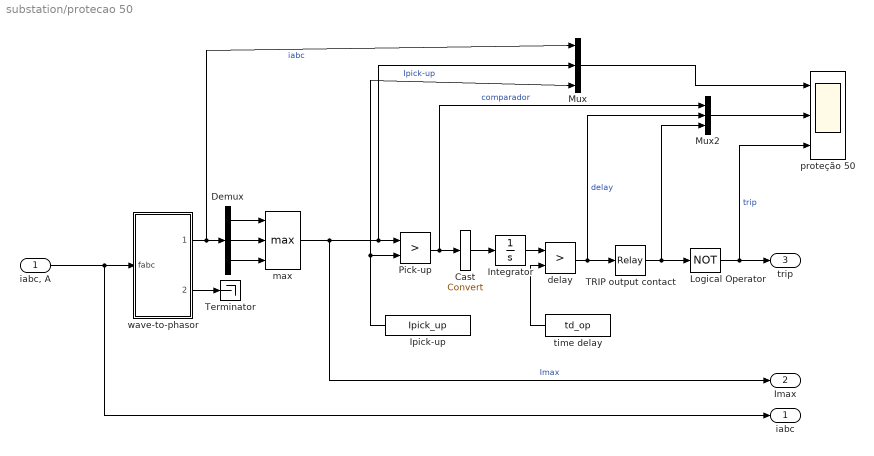
== system substation/protecao 50 ==
  "iabc, A" : Inport
  Cast : DataTypeConversion
  Demux : Demux  Outputs=3
  Integrator : Integrator
  Ipick-up : Constant  Value=Ipick_up
  Logical Operator : Logic  Operator=NOT  Inputs=1
  Mux : Mux  Inputs=3
  Mux2 : Mux  Inputs=3
  Pick-up : RelationalOperator  Operator=>  RndMeth=Nearest  InputSameDT=on
  TRIP output contact : Relay  OnSwitchValue=0.9999  OffSwitchValue=-1
  Terminator : Terminator
  delay : RelationalOperator  Operator=>  RndMeth=Nearest  InputSameDT=on
  max : MinMax  Function=max  Inputs=3
  proteção 50 : Scope  NumInputPorts=3
  time delay : Constant  Value=td_op
  wave-to-phasor : Subsystem
  iabc : Outport
  Imax : Outport  Port=2
  trip : Outport  Port=3
  wires:
  max/1 -> Imax/1, Mux/2, Pick-up/1  "Imax"
  TRIP output contact/1 -> Logical Operator/1, Mux2/3
  Mux2/1 -> proteção 50/2
  Cast/1 -> Integrator/1
  time delay/1 -> delay/2
  delay/1 -> TRIP output contact/1, Mux2/2  "delay"
  Logical Operator/1 -> trip/1, proteção 50/3  "trip"
  Mux/1 -> proteção 50/1
  Pick-up/1 -> Cast/1, Mux2/1  "comparador"
  Ipick-up/1 -> Mux/3, Pick-up/2  "Ipick-up"
  Integrator/1 -> delay/1
  Demux/1 -> max/1
  Demux/2 -> max/2
  Demux/3 -> max/3
  wave-to-phasor/1(|Fabc|) -> Mux/1, Demux/1  "iabc"
  "iabc, A"/1 -> wave-to-phasor/1(fabc), iabc/1
  wave-to-phasor/2(ang(Fabc)) -> Terminator/1

== system substation/Subsystem1/Subsystem ==
  Series RLC Branch1 : powerlib/Elements/Series RLC Branch  LConnTagsString=__new0  RConnTagsString=__new0  BranchType=RC  Resistance=1e9  Inductance=1e-3  SetiL0=off  InitialCurrent=0  Capacitance=1e-7  Setx0=off  InitialVoltage=0  Measurements=None
  Series RLC Branch2 : powerlib/Elements/Series RLC Branch  Commented=on  LConnTagsString=__new0  RConnTagsString=__new0  BranchType=RL  Resistance=1e9  Inductance=1e-3  SetiL0=off  InitialCurrent=0  Capacitance=1e-6  Setx0=off  InitialVoltage=0  Measurements=None
  A : PMIOPort  Side=Left
  a : PMIOPort  Port=2  Side=Right
  connections:
  Series RLC Branch2/RConn1 -- a/RConn1 -- Series RLC Branch1/RConn1
  Series RLC Branch2/LConn1 -- A/RConn1 -- Series RLC Branch1/LConn1

== system substation/Subsystem1/Subsystem1 ==
  Series RLC Branch1 : powerlib/Elements/Series RLC Branch  LConnTagsString=__new0  RConnTagsString=__new0  BranchType=RC  Resistance=1e9  Inductance=1e-3  SetiL0=off  InitialCurrent=0  Capacitance=1e-7  Setx0=off  InitialVoltage=0  Measurements=None
  Series RLC Branch2 : powerlib/Elements/Series RLC Branch  Commented=on  LConnTagsString=__new0  RConnTagsString=__new0  BranchType=RL  Resistance=1e9  Inductance=1e-3  SetiL0=off  InitialCurrent=0  Capacitance=1e-6  Setx0=off  InitialVoltage=0  Measurements=None
  A : PMIOPort  Side=Left
  a : PMIOPort  Port=2  Side=Right
  connections:
  Series RLC Branch1/LConn1 -- A/RConn1 -- Series RLC Branch2/LConn1
  Series RLC Branch1/RConn1 -- a/RConn1 -- Series RLC Branch2/RConn1

== system substation/Subsystem1/Subsystem3 ==
  Series RLC Branch1 : powerlib/Elements/Series RLC Branch  LConnTagsString=__new0  RConnTagsString=__new0  BranchType=RC  Resistance=1e9  Inductance=1e-3  SetiL0=off  InitialCurrent=0  Capacitance=1e-7  Setx0=off  InitialVoltage=0  Measurements=None
  Series RLC Branch2 : powerlib/Elements/Series RLC Branch  Commented=on  LConnTagsString=__new0  RConnTagsString=__new0  BranchType=RL  Resistance=1e9  Inductance=1e-3  SetiL0=off  InitialCurrent=0  Capacitance=1e-6  Setx0=off  InitialVoltage=0  Measurements=None
  A : PMIOPort  Side=Left
  a : PMIOPort  Port=2  Side=Right
  connections:
  Series RLC Branch2/RConn1 -- a/RConn1 -- Series RLC Branch1/RConn1
  Series RLC Branch2/LConn1 -- A/RConn1 -- Series RLC Branch1/LConn1

== system substation/Subsystem4/Subsystem ==
  Series RLC Branch1 : powerlib/Elements/Series RLC Branch  LConnTagsString=__new0  RConnTagsString=__new0  BranchType=RC  Resistance=1e9  Inductance=1e-3  SetiL0=off  InitialCurrent=0  Capacitance=1e-7  Setx0=off  InitialVoltage=0  Measurements=None
  Series RLC Branch2 : powerlib/Elements/Series RLC Branch  Commented=on  LConnTagsString=__new0  RConnTagsString=__new0  BranchType=RL  Resistance=1e9  Inductance=1e-3  SetiL0=off  InitialCurrent=0  Capacitance=1e-6  Setx0=off  InitialVoltage=0  Measurements=None
  A : PMIOPort  Side=Left
  a : PMIOPort  Port=2  Side=Right
  connections:
  Series RLC Branch1/LConn1 -- Series RLC Branch2/LConn1 -- A/RConn1
  Series RLC Branch1/RConn1 -- Series RLC Branch2/RConn1 -- a/RConn1

== system substation/Subsystem4/Subsystem1 ==
  Series RLC Branch1 : powerlib/Elements/Series RLC Branch  LConnTagsString=__new0  RConnTagsString=__new0  BranchType=RC  Resistance=1e9  Inductance=1e-3  SetiL0=off  InitialCurrent=0  Capacitance=1e-7  Setx0=off  InitialVoltage=0  Measurements=None
  Series RLC Branch2 : powerlib/Elements/Series RLC Branch  Commented=on  LConnTagsString=__new0  RConnTagsString=__new0  BranchType=RL  Resistance=1e9  Inductance=1e-3  SetiL0=off  InitialCurrent=0  Capacitance=1e-6  Setx0=off  InitialVoltage=0  Measurements=None
  A : PMIOPort  Side=Left
  a : PMIOPort  Port=2  Side=Right
  connections:
  Series RLC Branch2/RConn1 -- a/RConn1 -- Series RLC Branch1/RConn1
  Series RLC Branch2/LConn1 -- A/RConn1 -- Series RLC Branch1/LConn1

== system substation/Subsystem4/Subsystem3 ==
  Series RLC Branch1 : powerlib/Elements/Series RLC Branch  LConnTagsString=__new0  RConnTagsString=__new0  BranchType=RC  Resistance=1e9  Inductance=1e-3  SetiL0=off  InitialCurrent=0  Capacitance=1e-7  Setx0=off  InitialVoltage=0  Measurements=None
  Series RLC Branch2 : powerlib/Elements/Series RLC Branch  Commented=on  LConnTagsString=__new0  RConnTagsString=__new0  BranchType=RL  Resistance=1e9  Inductance=1e-3  SetiL0=off  InitialCurrent=0  Capacitance=1e-6  Setx0=off  InitialVoltage=0  Measurements=None
  A : PMIOPort  Side=Left
  a : PMIOPort  Port=2  Side=Right
  connections:
  Series RLC Branch1/LConn1 -- A/RConn1 -- Series RLC Branch2/LConn1
  Series RLC Branch1/RConn1 -- a/RConn1 -- Series RLC Branch2/RConn1

== system substation/Visualização/wave-to-phasor ==
  fabc : Inport
  Demux1 : Demux  Outputs=3
  Mux : Mux  Inputs=3
  Mux1 : Mux  Inputs=3
  RMS : powerlib_extras/Measurements/Fourier  f1=60  n=1
  RMS1 : powerlib_extras/Measurements/Fourier  f1=60  n=1
  RMS2 : powerlib_extras/Measurements/Fourier  f1=60  n=1
  |Fabc| : Outport
  ang(Fabc) : Outport  Port=2
  wires:
  Mux1/1 -> ang(Fabc)/1
  RMS/2 -> Mux1/1  "angIa"
  RMS1/2 -> Mux1/2
  RMS2/2 -> Mux1/3
  RMS2/1 -> Mux/3
  RMS1/1 -> Mux/2
  Mux/1 -> |Fabc|/1
  Demux1/3 -> RMS2/1
  Demux1/2 -> RMS1/1
  Demux1/1 -> RMS/1
  fabc/1 -> Demux1/1
  RMS/1 -> Mux/1  "|fa|"

== system substation/Visualização/wave-to-phasor1 ==
  fabc : Inport
  Demux1 : Demux  Outputs=3
  Mux : Mux  Inputs=3
  Mux1 : Mux  Inputs=3
  RMS : powerlib_extras/Measurements/Fourier  f1=60  n=1
  RMS1 : powerlib_extras/Measurements/Fourier  f1=60  n=1
  RMS2 : powerlib_extras/Measurements/Fourier  f1=60  n=1
  |Fabc| : Outport
  ang(Fabc) : Outport  Port=2
  wires:
  RMS/1 -> Mux/1  "|fa|"
  fabc/1 -> Demux1/1
  Demux1/1 -> RMS/1
  Demux1/2 -> RMS1/1
  Demux1/3 -> RMS2/1
  Mux/1 -> |Fabc|/1
  RMS1/1 -> Mux/2
  RMS2/1 -> Mux/3
  RMS2/2 -> Mux1/3
  RMS1/2 -> Mux1/2
  RMS/2 -> Mux1/1  "angIa"
  Mux1/1 -> ang(Fabc)/1

== system substation/Visualização1/wave-to-phasor ==
  fabc : Inport
  Demux1 : Demux  Outputs=3
  Mux : Mux  Inputs=3
  Mux1 : Mux  Inputs=3
  RMS : powerlib_extras/Measurements/Fourier  f1=60  n=1
  RMS1 : powerlib_extras/Measurements/Fourier  f1=60  n=1
  RMS2 : powerlib_extras/Measurements/Fourier  f1=60  n=1
  |Fabc| : Outport
  ang(Fabc) : Outport  Port=2
  wires:
  RMS/1 -> Mux/1  "|fa|"
  fabc/1 -> Demux1/1
  Demux1/1 -> RMS/1
  Demux1/2 -> RMS1/1
  Demux1/3 -> RMS2/1
  Mux/1 -> |Fabc|/1
  RMS1/1 -> Mux/2
  RMS2/1 -> Mux/3
  RMS2/2 -> Mux1/3
  RMS1/2 -> Mux1/2
  RMS/2 -> Mux1/1  "angIa"
  Mux1/1 -> ang(Fabc)/1

== system substation/Visualização1/wave-to-phasor1 ==
  fabc : Inport
  Demux1 : Demux  Outputs=3
  Mux : Mux  Inputs=3
  Mux1 : Mux  Inputs=3
  RMS : powerlib_extras/Measurements/Fourier  f1=60  n=1
  RMS1 : powerlib_extras/Measurements/Fourier  f1=60  n=1
  RMS2 : powerlib_extras/Measurements/Fourier  f1=60  n=1
  |Fabc| : Outport
  ang(Fabc) : Outport  Port=2
  wires:
  Mux1/1 -> ang(Fabc)/1
  RMS/2 -> Mux1/1  "angIa"
  RMS1/2 -> Mux1/2
  RMS2/2 -> Mux1/3
  RMS2/1 -> Mux/3
  RMS1/1 -> Mux/2
  Mux/1 -> |Fabc|/1
  Demux1/3 -> RMS2/1
  Demux1/2 -> RMS1/1
  Demux1/1 -> RMS/1
  fabc/1 -> Demux1/1
  RMS/1 -> Mux/1  "|fa|"

== system substation/Visualização2/wave-to-phasor ==
  fabc : Inport
  Demux1 : Demux  Outputs=3
  Mux : Mux  Inputs=3
  Mux1 : Mux  Inputs=3
  RMS : powerlib_extras/Measurements/Fourier  f1=60  n=1
  RMS1 : powerlib_extras/Measurements/Fourier  f1=60  n=1
  RMS2 : powerlib_extras/Measurements/Fourier  f1=60  n=1
  |Fabc| : Outport
  ang(Fabc) : Outport  Port=2
  wires:
  Mux1/1 -> ang(Fabc)/1
  RMS/2 -> Mux1/1  "angIa"
  RMS1/2 -> Mux1/2
  RMS2/2 -> Mux1/3
  RMS2/1 -> Mux/3
  RMS1/1 -> Mux/2
  Mux/1 -> |Fabc|/1
  Demux1/3 -> RMS2/1
  Demux1/2 -> RMS1/1
  Demux1/1 -> RMS/1
  fabc/1 -> Demux1/1
  RMS/1 -> Mux/1  "|fa|"

== system substation/Visualização2/wave-to-phasor1 ==
  fabc : Inport
  Demux1 : Demux  Outputs=3
  Mux : Mux  Inputs=3
  Mux1 : Mux  Inputs=3
  RMS : powerlib_extras/Measurements/Fourier  f1=60  n=1
  RMS1 : powerlib_extras/Measurements/Fourier  f1=60  n=1
  RMS2 : powerlib_extras/Measurements/Fourier  f1=60  n=1
  |Fabc| : Outport
  ang(Fabc) : Outport  Port=2
  wires:
  RMS/1 -> Mux/1  "|fa|"
  fabc/1 -> Demux1/1
  Demux1/1 -> RMS/1
  Demux1/2 -> RMS1/1
  Demux1/3 -> RMS2/1
  Mux/1 -> |Fabc|/1
  RMS1/1 -> Mux/2
  RMS2/1 -> Mux/3
  RMS2/2 -> Mux1/3
  RMS1/2 -> Mux1/2
  RMS/2 -> Mux1/1  "angIa"
  Mux1/1 -> ang(Fabc)/1

== system substation/Visualização3/wave-to-phasor ==
  fabc : Inport
  Demux1 : Demux  Outputs=3
  Mux : Mux  Inputs=3
  Mux1 : Mux  Inputs=3
  RMS : powerlib_extras/Measurements/Fourier  f1=60  n=1
  RMS1 : powerlib_extras/Measurements/Fourier  f1=60  n=1
  RMS2 : powerlib_extras/Measurements/Fourier  f1=60  n=1
  |Fabc| : Outport
  ang(Fabc) : Outport  Port=2
  wires:
  RMS/1 -> Mux/1  "|fa|"
  fabc/1 -> Demux1/1
  Demux1/1 -> RMS/1
  Demux1/2 -> RMS1/1
  Demux1/3 -> RMS2/1
  Mux/1 -> |Fabc|/1
  RMS1/1 -> Mux/2
  RMS2/1 -> Mux/3
  RMS2/2 -> Mux1/3
  RMS1/2 -> Mux1/2
  RMS/2 -> Mux1/1  "angIa"
  Mux1/1 -> ang(Fabc)/1

== system substation/Visualização3/wave-to-phasor1 ==
  fabc : Inport
  Demux1 : Demux  Outputs=3
  Mux : Mux  Inputs=3
  Mux1 : Mux  Inputs=3
  RMS : powerlib_extras/Measurements/Fourier  f1=60  n=1
  RMS1 : powerlib_extras/Measurements/Fourier  f1=60  n=1
  RMS2 : powerlib_extras/Measurements/Fourier  f1=60  n=1
  |Fabc| : Outport
  ang(Fabc) : Outport  Port=2
  wires:
  Mux1/1 -> ang(Fabc)/1
  RMS/2 -> Mux1/1  "angIa"
  RMS1/2 -> Mux1/2
  RMS2/2 -> Mux1/3
  RMS2/1 -> Mux/3
  RMS1/1 -> Mux/2
  Mux/1 -> |Fabc|/1
  Demux1/3 -> RMS2/1
  Demux1/2 -> RMS1/1
  Demux1/1 -> RMS/1
  fabc/1 -> Demux1/1
  RMS/1 -> Mux/1  "|fa|"

== system substation/Visualização4/wave-to-phasor ==
  fabc : Inport
  Demux1 : Demux  Outputs=3
  Mux : Mux  Inputs=3
  Mux1 : Mux  Inputs=3
  RMS : powerlib_extras/Measurements/Fourier  f1=60  n=1
  RMS1 : powerlib_extras/Measurements/Fourier  f1=60  n=1
  RMS2 : powerlib_extras/Measurements/Fourier  f1=60  n=1
  |Fabc| : Outport
  ang(Fabc) : Outport  Port=2
  wires:
  Mux1/1 -> ang(Fabc)/1
  RMS/2 -> Mux1/1  "angIa"
  RMS1/2 -> Mux1/2
  RMS2/2 -> Mux1/3
  RMS2/1 -> Mux/3
  RMS1/1 -> Mux/2
  Mux/1 -> |Fabc|/1
  Demux1/3 -> RMS2/1
  Demux1/2 -> RMS1/1
  Demux1/1 -> RMS/1
  fabc/1 -> Demux1/1
  RMS/1 -> Mux/1  "|fa|"

== system substation/Visualização4/wave-to-phasor1 ==
  fabc : Inport
  Demux1 : Demux  Outputs=3
  Mux : Mux  Inputs=3
  Mux1 : Mux  Inputs=3
  RMS : powerlib_extras/Measurements/Fourier  f1=60  n=1
  RMS1 : powerlib_extras/Measurements/Fourier  f1=60  n=1
  RMS2 : powerlib_extras/Measurements/Fourier  f1=60  n=1
  |Fabc| : Outport
  ang(Fabc) : Outport  Port=2
  wires:
  RMS/1 -> Mux/1  "|fa|"
  fabc/1 -> Demux1/1
  Demux1/1 -> RMS/1
  Demux1/2 -> RMS1/1
  Demux1/3 -> RMS2/1
  Mux/1 -> |Fabc|/1
  RMS1/1 -> Mux/2
  RMS2/1 -> Mux/3
  RMS2/2 -> Mux1/3
  RMS1/2 -> Mux1/2
  RMS/2 -> Mux1/1  "angIa"
  Mux1/1 -> ang(Fabc)/1
